simulink model "accController"  (R2022b)
settings: Solver=FixedStepAuto  StartTime=0.0  StopTime=120  FixedStep=tSample  RelTol=1e-3  EnableMultiTasking=on
PreLoadFcn:
  | if exist('tl_preloadfcn','file'), tl_preloadfcn(gcs,'22.1.0.27'); end
PostLoadFcn:
  | if exist('tl_postloadfcn','file'), tl_postloadfcn(gcs,'22.1.0.27'); end
InitFcn:
  | if exist('tlds_init','file'), tlds_init(gcs); end
StartFcn:
  | if exist('tlds_start','file'), tlds_start(gcs); end
StopFcn:
  | if exist('tlds_stop','file'), tlds_stop(gcs); end
model workspace (MAT data in the model file):
  obs_1 = 1
  obs_10 = 1
  obs_11 = 1
  obs_12 = 1
  obs_13 = 1
  obs_14 = 1
  obs_15 = 1
  obs_16 = 1
  obs_17 = 1
  obs_18 = 1
  obs_19 = 1
  obs_2 = 1
  obs_20 = 1
  obs_21 = 1
  obs_22 = 1
  obs_23 = 1
  obs_24 = 1
  obs_25 = 1
  obs_26 = 1
  obs_27 = 1
  obs_28 = 1
  obs_29 = 1
  obs_3 = 1
  obs_30 = 1
  obs_31 = 1
  obs_32 = 1
  obs_4 = 1
  obs_5 = 1
  obs_6 = 1
  obs_7 = 1
  obs_8 = 1
  obs_9 = 1
values from neighbouring files (symbols this model uses):
  pLutAccelMagnitude = [0, 0.1, 0.2, 0.3, 0.4, 0.5, 0.6, 0.7, 0.8, 0.9, 1,                        2.5, 3, 3.5, 4, 4.5, 5, 8, 12, 20]    [start.m]
  pLutAccelnSeverity = [0, 0.005, 0.05, 0.1, 0.15, 0.2, 0.3, 0.4, 0.6, 1, 3,                        5, 10, 17, 24, 32, 45, 60, 75, 100]    [start.m]
  pMaxAccAcceleration = 1.5    [start.m]
  pMaxAccDeacceleration = -1.5    [start.m]
  pMaxOperatingSpeed = 180    [start.m]
  pMinOperatingSpeed = 30    [start.m]
  tSample = 0.01    [start.m]
undefined symbols (not defined in the file or in its folder): Pedal, sigbuilder_block, vehicleDistanceRange
libraries: tllib x7
(part 1 of 5)
PreSaveFcn:
  | if exist('tl_presavefcn','file'), tl_presavefcn(gcs); end
CloseFcn:
  | if exist('tl_closefcn','file'), tl_closefcn(gcs); end
settings Model: TL_MAIN_DATA={'date',739002.69656854169,'advcodeopt',{'ExtendedBlockComments';'true'}}  DS_PROJECTFILE=accController.dd  TLVersion=22.1.0.27  TL_GLOBAL_LOGGING_MODE=4  PauseTimes=80.79  NumberOfSteps=100  Creator=developer  LastModifiedBy=developer
settings SolverCC: AlgebraicLoopSolver=TrustRegion
settings DataIOCC: LimitDataPoints=on  SaveFormat=Array  ReturnWorkspaceOutputs=off
settings OptimizationCC: BlockReduction=off  ConditionallyExecuteInputs=off  OptimizeBlockIOStorage=off  BufferReuse=off  GlobalBufferReuse=off  ExpressionFolding=off  LocalBlockOutputs=off  LifeSpan=inf  OptimizeDataStoreBuffers=off  BusAssignmentInplaceUpdate=off
settings DebuggingCC: UnconnectedInputMsg=warning  UnconnectedOutputMsg=warning  UnconnectedLineMsg=warning  BusObjectLabelMismatch=error  StrictBusMsg=ErrorOnBusTreatedAsVector  NonBusSignalsTreatedAsBus=error  SFUnexpectedBacktrackingDiag=warning  SFNoUnconditionalDefaultTransitionDiag=warning  SFMachineParentedDataDiag=warning  ArithmeticOperatorsInVariantConditions=warning
settings HardwareCC: ProdBitPerPointer=32  ProdBitPerSizeT=32  ProdBitPerPtrDiffT=32  ProdLargestAtomicFloat=None  ProdIntDivRoundTo=Undefined  ProdEndianess=Unspecified  ProdWordSize=32  ProdHWDeviceType=32-bit Generic
settings ModelReferenceCC: EnableRefExpFcnMdlSchedulingChecks=on  PropagateSignalLabelsOutOfModel=off
settings SFSimCC: SimUseLocalCustomCode=off  CustomCodeUndefinedFunction=UseInterfaceOnly
settings RTWCC: RTWUseLocalCustomCode=off
settings CodeAppCC: StateflowObjectComments=on
settings GRTTargetCC: TargetLangStandard=C89/C90 (ANSI)
settings ConfigComp: CovMetricSettings=dw  CovSaveCumulativeToWorkspaceVar=on  CovSaveSingleToWorkspaceVar=on  CovExternalEMLEnable=off

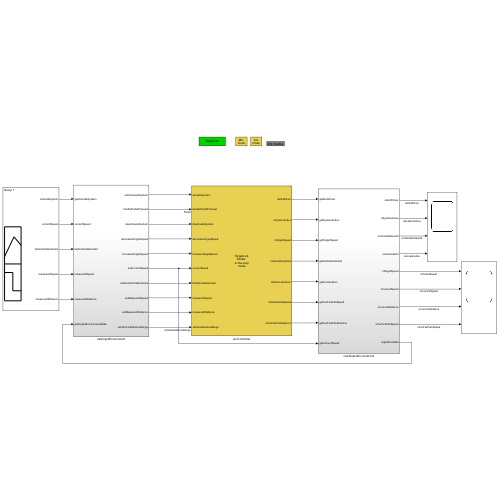
[thumbnail: Simulink's stored preview of the top-level diagram]
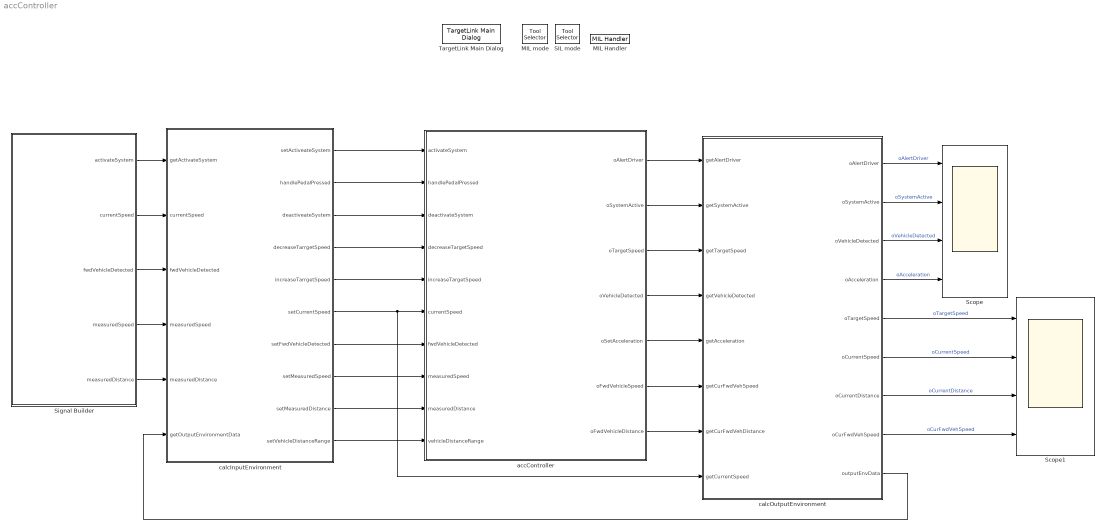
== system accController ==
  MIL Handler : tllib/MIL Handler  data={'date',730486}
      settings: SourceProductName=dSPACE TargetLink common blockset
  MIL mode : tllib/Tool Selector  Description=MIL\nmode  data={'date',730486}
      settings: SourceProductName=dSPACE TargetLink common blockset
  SIL mode : tllib/Tool Selector  Description=SIL\nmode  data={'date',730486}
      settings: SourceProductName=dSPACE TargetLink common blockset
  Scope : Scope  NumInputPorts=4
  Scope1 : Scope  NumInputPorts=4
  Signal Builder : Subsystem  Tag=STV Subsys  LoadFcn=sigbuilder_block('load');  StartFcn=sigbuilder_block('start');  StopFcn=sigbuilder_block('stop');  ClipboardFcn=sigbuilder_block('clipboard');  mask(Sigbuilder block){tuvar=[0:10]}
      mask help: Simulink:masks:SigbuilderBlock_MD
      mask init:
      | if ~strcmp(get_param(bdroot(gcbh),'SimulationStatus'),'stopped') tuvar = sigbuilder_block('maskInit'); end
      settings: CopyFcn=sigbuilder_block('copy');  DeleteFcn=sigbuilder_block('delete');  ModelCloseFcn=sigbuilder_block('modelClose');  PreSaveFcn=sigbuilder_block('preSave');  PauseFcn=sigbuilder_block('pause');  ContinueFcn=sigbuilder_block('continue');  NameChangeFcn=sigbuilder_block('namechange');  OpenFcn=sigbuilder_block('open',[133.5 114.75 1037.25 597 ]);  CloseFcn=sigbuilder_block('close');
      mask Display: plot(0, 0, 100, 100,[2, 2, 32, 32, 2], [68, 8, 8, 68, 68],[32, 2], [38, 38], [32, 19, 2],[53, 60, 44], [32, 17, 17, 2],[16, 16, 31, 31]);txt = getActiveGroup(gcbh);text(2, 100, txt,'verticalAlignment', 'top');
  TargetLink Main Dialog : tllib/TargetLink Main Dialog  data=[]
      settings: SourceProductName=dSPACE TargetLink common blockset
  accController : Subsystem  Tag=TargetLink Simulation Frame  mask(TL_SimFrame){}
      settings: CopyFcn=if exist('tl_copyfcn','file'), tl_copyfcn(gcbh); end  NameChangeFcn=if exist('tl_framenamechangefcn','file'), tl_framenamechangefcn(gcbh); end
      settings: OpenFcn=|
      | if exist('open_tlsubsystem','file')
      |    open_tlsubsystem(gcbh);
      | else
      |    tlsubsystem = ...
      |       find_system(gcb, ...
      |       'LookUnderMasks','on', ...
      |       'FollowLinks','on', ...
      |       'Tag','MIL Subsystem');
      |    open_system(tlsubsystem);
      | end
      mask Display: disp('TargetLink\nModel-\nin-the-loop\nmode')
  calcInputEnvironment : Subsystem
  calcOutputEnvironment : Subsystem
  wires:
  calcInputEnvironment/2(handlePedalPressed) -> accController/2(handlePedalPressed)
  calcInputEnvironment/10(setVehicleDistanceRange) -> accController/10(vehicleDistanceRange)
  accController/1(oAlertDriver) -> calcOutputEnvironment/1(getAlertDriver)
  calcInputEnvironment/9(setMeasuredDistance) -> accController/9(measuredDistance)
  accController/4(oVehicleDetected) -> calcOutputEnvironment/4(getVehicleDetected)
  calcInputEnvironment/6(setCurrentSpeed) -> calcOutputEnvironment/8(getCurrentSpeed), accController/6(currentSpeed)
  accController/5(oSetAcceleration) -> calcOutputEnvironment/5(getAcceleration)
  accController/6(oFwdVehicleSpeed) -> calcOutputEnvironment/6(getCurFwdVehSpeed)
  accController/7(oFwdVehicleDistance) -> calcOutputEnvironment/7(getCurFwdVehDistance)
  Signal Builder/1(activateSystem) -> calcInputEnvironment/1(getActivateSystem)
  Signal Builder/2(currentSpeed) -> calcInputEnvironment/2(currentSpeed)
  Signal Builder/3(fwdVehicleDetected) -> calcInputEnvironment/3(fwdVehicleDetected)
  Signal Builder/4(measuredSpeed) -> calcInputEnvironment/4(measuredSpeed)
  Signal Builder/5(measuredDistance) -> calcInputEnvironment/5(measuredDistance)
  accController/2(oSystemActive) -> calcOutputEnvironment/2(getSystemActive)
  accController/3(oTargetSpeed) -> calcOutputEnvironment/3(getTargetSpeed)
  calcInputEnvironment/3(deactiveateSystem) -> accController/3(deactivateSystem)
  calcInputEnvironment/4(decreaseTarrgetSpeed) -> accController/4(decreaseTargetSpeed)
  calcInputEnvironment/5(increaseTarrgetSpeed) -> accController/5(increaseTargetSpeed)
  calcOutputEnvironment/9(outputEnvData) -> calcInputEnvironment/6(getOutputEnvironmentData)
  calcInputEnvironment/7(setFwdVehicleDetected) -> accController/7(fwdVehicleDetected)
  calcInputEnvironment/8(setMeasuredSpeed) -> accController/8(measuredSpeed)
  calcInputEnvironment/1(setActiveateSystem) -> accController/1(activateSystem)
  calcOutputEnvironment/1(oAlertDriver) -> Scope/1  "oAlertDriver"
  calcOutputEnvironment/2(oSystemActive) -> Scope/2  "oSystemActive"
  calcOutputEnvironment/3(oVehicleDetected) -> Scope/3  "oVehicleDetected"
  calcOutputEnvironment/5(oTargetSpeed) -> Scope1/1  "oTargetSpeed"
  calcOutputEnvironment/6(oCurrentSpeed) -> Scope1/2  "oCurrentSpeed"
  calcOutputEnvironment/7(oCurrentDistance) -> Scope1/3  "oCurrentDistance"
  calcOutputEnvironment/8(oCurFwdVehSpeed) -> Scope1/4  "oCurFwdVehSpeed"
  calcOutputEnvironment/4(oAcceleration) -> Scope/4  "oAcceleration"

== system accController/Signal Builder ==
  Demux : Demux  Tag=STV Demux  Outputs=5
      settings: DisplayOption=none
  FromWs : FromWorkspace  Tag=STV FromWs  VariableName=tuvar
      SigBuilderData=|
      | common.afterFinalStr = 'Extrapolate'
      | common.sampleTime = 0
      | dataSet.timeRange = [0 120]
      | dataSet.name = 'Group 1'
      | sbobj.Groups.Name = 'Group 1'
      | sbobj.Groups.Signals(1).Name = 'activateSystem'
      | sbobj.Groups.Signals(1).XData = [0 12 12 13 13 120]
      | sbobj.Groups.Signals(1).YData = [0 0 1 1 0 0]
      | sbobj.Groups.Signals(2).Name = 'currentSpeed'
      | sbobj.Groups.Signals(2).XData = [0 12 120]
      | sbobj.Groups.Signals(2).YData = [0 135 135]
      | sbobj.Groups.Signals(3).Name = 'fwdVehicleDetected'
      | sbobj.Groups.Signals(3).XData = [0 20 20 120]
      | sbobj.Groups.Signals(3).YData = [0 0 1 1]
      | sbobj.Groups.Signals(4).Name = 'measuredSpeed'
      | sbobj.Groups.Signals(4).XData = [0 20 120]
      | sbobj.Groups.Signals(4).YData = [0 100 100]
      | sbobj.Groups.Signals(5).Name = 'measuredDistance'
      | sbobj.Groups.Signals(5).XData = [0 20 20 60 120]
      | sbobj.Groups.Signals(5).YData = [0 0 144 40 40]
      | sbobj.Groups.TimeRange = [0 120]
  activateSystem : Outport  Tag=STV Outport
  currentSpeed : Outport  Tag=STV Outport  Port=2
  fwdVehicleDetected : Outport  Tag=STV Outport  Port=3
  measuredSpeed : Outport  Tag=STV Outport  Port=4
  measuredDistance : Outport  Tag=STV Outport  Port=5
  wires:
  FromWs/1 -> Demux/1
  Demux/1 -> activateSystem/1
  Demux/2 -> currentSpeed/1
  Demux/3 -> fwdVehicleDetected/1
  Demux/4 -> measuredSpeed/1
  Demux/5 -> measuredDistance/1

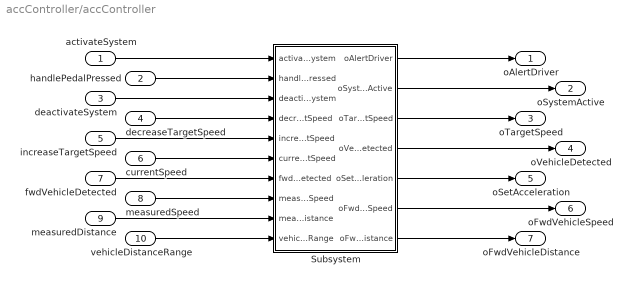
== system accController/accController ==
  activateSystem : Inport
  handlePedalPressed : Inport  Port=2  OutDataTypeStr=Enum: Pedal
  deactivateSystem : Inport  Port=3
  decreaseTargetSpeed : Inport  Port=4
  increaseTargetSpeed : Inport  Port=5
  currentSpeed : Inport  Port=6
  fwdVehicleDetected : Inport  Port=7
  measuredSpeed : Inport  Port=8
  measuredDistance : Inport  Port=9
  vehicleDistanceRange : Inport  Port=10  OutDataTypeStr=Enum: vehicleDistanceRange
  Subsystem : Subsystem  Tag=struct('sfcnName','accController_sf','subFunction','','srcSubsystem','')  mask(TL_Enable){}
      settings: OpenFcn=warndlg(get_param(gcb,'MaskHelp'),'Serious Warning');
      mask Help: This subsystem keeps the TargetLink subsystem (subsystem with TargetLink blocks for production code generation), and is needed for the TargetLink simulation frame to work properly. DO NOT DELETE OR MODIFY IT!
  oAlertDriver : Outport
  oSystemActive : Outport  Port=2
  oTargetSpeed : Outport  Port=3
  oVehicleDetected : Outport  Port=4
  oSetAcceleration : Outport  Port=5
  oFwdVehicleSpeed : Outport  Port=6
  oFwdVehicleDistance : Outport  Port=7
  wires:
  activateSystem/1 -> Subsystem/1(activateSystem)
  handlePedalPressed/1 -> Subsystem/2(handlePedalPressed)
  deactivateSystem/1 -> Subsystem/3(deactivateSystem)
  decreaseTargetSpeed/1 -> Subsystem/4(decreaseTargetSpeed)
  increaseTargetSpeed/1 -> Subsystem/5(increaseTargetSpeed)
  currentSpeed/1 -> Subsystem/6(currentSpeed)
  fwdVehicleDetected/1 -> Subsystem/7(fwdVehicleDetected)
  measuredSpeed/1 -> Subsystem/8(measuredSpeed)
  measuredDistance/1 -> Subsystem/9(measuredDistance)
  vehicleDistanceRange/1 -> Subsystem/10(vehicleDistanceRange)
  Subsystem/1(oAlertDriver) -> oAlertDriver/1
  Subsystem/2(oSystemActive) -> oSystemActive/1
  Subsystem/3(oTargetSpeed) -> oTargetSpeed/1
  Subsystem/4(oVehicleDetected) -> oVehicleDetected/1
  Subsystem/5(oSetAcceleration) -> oSetAcceleration/1
  Subsystem/6(oFwdVehicleSpeed) -> oFwdVehicleSpeed/1
  Subsystem/7(oFwdVehicleDistance) -> oFwdVehicleDistance/1

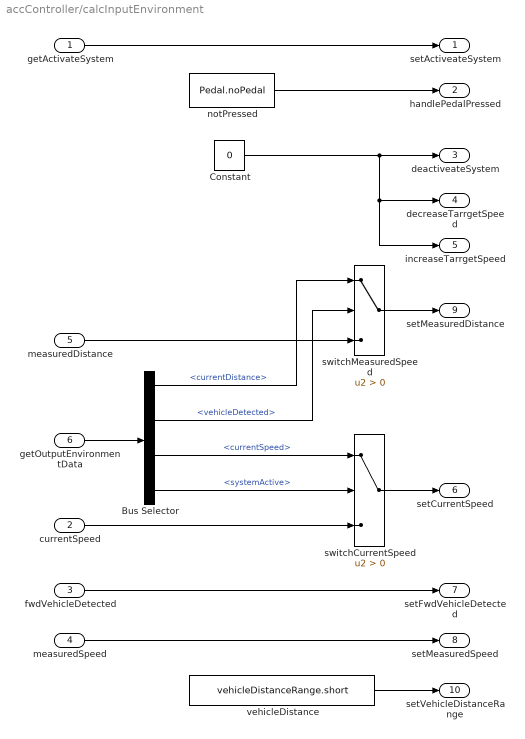
== system accController/calcInputEnvironment ==
  getActivateSystem : Inport
  currentSpeed : Inport  Port=2
  fwdVehicleDetected : Inport  Port=3
  measuredSpeed : Inport  Port=4
  measuredDistance : Inport  Port=5
  getOutputEnvironmentData : Inport  Port=6
  Bus Selector : BusSelector  OutputSignals=currentDistance,vehicleDetected,currentSpeed,systemActive
  Constant : Constant  Value=0
  notPressed : Constant  Value=Pedal.noPedal  OutDataTypeStr=Enum: Pedal
  switchCurrentSpeed : Switch  Criteria=u2 > Threshold  SaturateOnIntegerOverflow=off  InputSameDT=off
  switchMeasuredSpeed : Switch  Criteria=u2 > Threshold  SaturateOnIntegerOverflow=off  InputSameDT=off
  vehicleDistance : Constant  Value=vehicleDistanceRange.short  OutDataTypeStr=Enum: vehicleDistanceRange
  setActiveateSystem : Outport
  handlePedalPressed : Outport  Port=2
  deactiveateSystem : Outport  Port=3
  decreaseTarrgetSpeed : Outport  Port=4
  increaseTarrgetSpeed : Outport  Port=5
  setCurrentSpeed : Outport  Port=6
  setFwdVehicleDetected : Outport  Port=7
  setMeasuredSpeed : Outport  Port=8
  setMeasuredDistance : Outport  Port=9
  setVehicleDistanceRange : Outport  Port=10
  wires:
  getActivateSystem/1 -> setActiveateSystem/1
  vehicleDistance/1 -> setVehicleDistanceRange/1
  notPressed/1 -> handlePedalPressed/1
  Constant/1 -> increaseTarrgetSpeed/1, decreaseTarrgetSpeed/1, deactiveateSystem/1
  getOutputEnvironmentData/1 -> Bus Selector/1
  switchCurrentSpeed/1 -> setCurrentSpeed/1
  Bus Selector/4 -> switchCurrentSpeed/2  "<systemActive>"
  Bus Selector/3 -> switchCurrentSpeed/1  "<currentSpeed>"
  currentSpeed/1 -> switchCurrentSpeed/3
  fwdVehicleDetected/1 -> setFwdVehicleDetected/1
  Bus Selector/1 -> switchMeasuredSpeed/1  "<currentDistance>"
  Bus Selector/2 -> switchMeasuredSpeed/2  "<vehicleDetected>"
  measuredDistance/1 -> switchMeasuredSpeed/3
  switchMeasuredSpeed/1 -> setMeasuredDistance/1
  measuredSpeed/1 -> setMeasuredSpeed/1

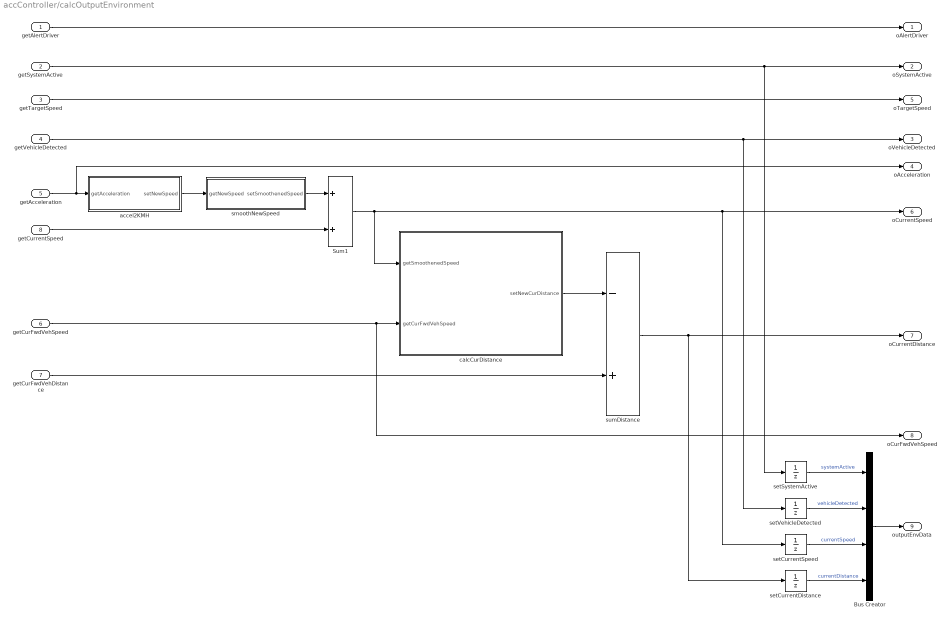
== system accController/calcOutputEnvironment ==
  getAlertDriver : Inport
  getSystemActive : Inport  Port=2
  getTargetSpeed : Inport  Port=3
  getVehicleDetected : Inport  Port=4
  getAcceleration : Inport  Port=5
  getCurFwdVehSpeed : Inport  Port=6
  getCurFwdVehDistance : Inport  Port=7
  getCurrentSpeed : Inport  Port=8
  Bus Creator : BusCreator  Inputs=4
  Sum1 : Sum
  accel2KMH : Subsystem
  calcCurDistance : Subsystem
  setCurrentDistance : UnitDelay  SampleTime=-1  HasFrameUpgradeWarning=on
  setCurrentSpeed : UnitDelay  SampleTime=-1  HasFrameUpgradeWarning=on
  setSystemActive : UnitDelay  SampleTime=-1  HasFrameUpgradeWarning=on
  setVehicleDetected : UnitDelay  SampleTime=-1  HasFrameUpgradeWarning=on
  smoothNewSpeed : Subsystem
  sumDistance : Sum  Inputs=-+
  oAlertDriver : Outport
  oSystemActive : Outport  Port=2
  oVehicleDetected : Outport  Port=3
  oAcceleration : Outport  Port=4
  oTargetSpeed : Outport  Port=5
  oCurrentSpeed : Outport  Port=6
  oCurrentDistance : Outport  Port=7
  oCurFwdVehSpeed : Outport  Port=8
  outputEnvData : Outport  Port=9
  wires:
  getAcceleration/1 -> oAcceleration/1, accel2KMH/1(getAcceleration)
  accel2KMH/1(setNewSpeed) -> smoothNewSpeed/1(getNewSpeed)
  smoothNewSpeed/1(setSmoothenedSpeed) -> Sum1/1
  Sum1/1 -> calcCurDistance/1(getSmoothenedSpeed), setCurrentSpeed/1, oCurrentSpeed/1
  getCurrentSpeed/1 -> Sum1/2
  getCurFwdVehSpeed/1 -> oCurFwdVehSpeed/1, calcCurDistance/2(getCurFwdVehSpeed)
  calcCurDistance/1(setNewCurDistance) -> sumDistance/1
  getCurFwdVehDistance/1 -> sumDistance/2
  sumDistance/1 -> oCurrentDistance/1, setCurrentDistance/1
  getAlertDriver/1 -> oAlertDriver/1
  getTargetSpeed/1 -> oTargetSpeed/1
  getSystemActive/1 -> oSystemActive/1, setSystemActive/1
  getVehicleDetected/1 -> oVehicleDetected/1, setVehicleDetected/1
  Bus Creator/1 -> outputEnvData/1
  setSystemActive/1 -> Bus Creator/1  "systemActive"
  setVehicleDetected/1 -> Bus Creator/2  "vehicleDetected"
  setCurrentSpeed/1 -> Bus Creator/3  "currentSpeed"
  setCurrentDistance/1 -> Bus Creator/4  "currentDistance"

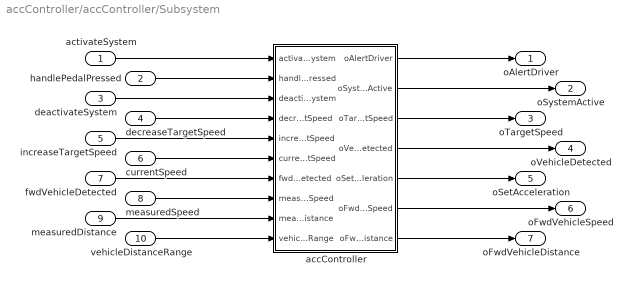
== system accController/accController/Subsystem ==
  activateSystem : Inport
  handlePedalPressed : Inport  Port=2
  deactivateSystem : Inport  Port=3
  decreaseTargetSpeed : Inport  Port=4
  increaseTargetSpeed : Inport  Port=5
  currentSpeed : Inport  Port=6
  fwdVehicleDetected : Inport  Port=7
  measuredSpeed : Inport  Port=8
  measuredDistance : Inport  Port=9
  vehicleDistanceRange : Inport  Port=10
  accController : Subsystem  Tag=MIL Subsystem  Description=a  LoadFcn=|
      | if exist('TargetLink.SimFrameHandler.TLSubsystem','class')
      |     TargetLink.SimFrameHandler.TLSubsystem.CreateWatchDog(gcbh);
      | end
      settings: AttributesFormatString=$ V-ECU simulation $\nUUID = ac35bcf0-8bf8-4691-a732-4e92aa29c2f7\nXCP-Port = \n  CopyFcn=if exist('tl_copyfcn','file'), tl_copyfcn(gcbh); end  NameChangeFcn=if exist('tl_namechangefcn','file'), tl_namechangefcn(gcbh); end  DestroyFcn=if exist('update_tl_main_dlg','file'), update_tl_main_dlg('TL_subs_display'); end
  oAlertDriver : Outport
  oSystemActive : Outport  Port=2
  oTargetSpeed : Outport  Port=3
  oVehicleDetected : Outport  Port=4
  oSetAcceleration : Outport  Port=5
  oFwdVehicleSpeed : Outport  Port=6
  oFwdVehicleDistance : Outport  Port=7
  wires:
  activateSystem/1 -> accController/1(activateSystem)
  handlePedalPressed/1 -> accController/2(handlePedalPressed)
  deactivateSystem/1 -> accController/3(deactivateSystem)
  decreaseTargetSpeed/1 -> accController/4(decreaseTargetSpeed)
  increaseTargetSpeed/1 -> accController/5(increaseTargetSpeed)
  currentSpeed/1 -> accController/6(currentSpeed)
  fwdVehicleDetected/1 -> accController/7(fwdVehicleDetected)
  measuredSpeed/1 -> accController/8(measuredSpeed)
  measuredDistance/1 -> accController/9(measuredDistance)
  vehicleDistanceRange/1 -> accController/10(vehicleDistanceRange)
  accController/1(oAlertDriver) -> oAlertDriver/1
  accController/2(oSystemActive) -> oSystemActive/1
  accController/3(oTargetSpeed) -> oTargetSpeed/1
  accController/4(oVehicleDetected) -> oVehicleDetected/1
  accController/5(oSetAcceleration) -> oSetAcceleration/1
  accController/6(oFwdVehicleSpeed) -> oFwdVehicleSpeed/1
  accController/7(oFwdVehicleDistance) -> oFwdVehicleDistance/1

== system accController/calcOutputEnvironment/accel2KMH ==
  getAcceleration : Inport
  acc2Speed : Product
  acc2Speed1 : Product
  ms2kmh : Constant  Value=3.6
  samplingTimeDiv : Constant  Value=tSample
  setNewSpeed : Outport
  wires:
  getAcceleration/1 -> acc2Speed/1
  samplingTimeDiv/1 -> acc2Speed/2
  acc2Speed/1 -> acc2Speed1/1
  ms2kmh/1 -> acc2Speed1/2
  acc2Speed1/1 -> setNewSpeed/1

== system accController/calcOutputEnvironment/calcCurDistance ==
  getSmoothenedSpeed : Inport
  getCurFwdVehSpeed : Inport  Port=2
  diffSpeed : Sum  Inputs=+-
  kmh2ms : Constant  Value=3.6
  kmh2msDiv : Product  Inputs=*/
  runDistance : Product
  samplingTimeDiv : Constant  Value=tSample
  setNewCurDistance : Outport
  wires:
  getSmoothenedSpeed/1 -> diffSpeed/1
  diffSpeed/1 -> kmh2msDiv/1
  kmh2ms/1 -> kmh2msDiv/2
  kmh2msDiv/1 -> runDistance/1
  samplingTimeDiv/1 -> runDistance/2
  runDistance/1 -> setNewCurDistance/1
  getCurFwdVehSpeed/1 -> diffSpeed/2

== system accController/calcOutputEnvironment/smoothNewSpeed ==
  getNewSpeed : Inport
  Abs : Abs  SaturateOnIntegerOverflow=off
  Sum : Sum
  chSpdThreshhold : Constant
  chSpeed : Switch  Criteria=u2 > Threshold  SaturateOnIntegerOverflow=off  InputSameDT=off
  changeSpeed : RelationalOperator  OutDataTypeStr=boolean  InputSameDT=off
  keepSpeed : Constant  Value=0
  resetUnitDelay : Switch  Threshold=1  SaturateOnIntegerOverflow=off  InputSameDT=off
  resetValue : Constant  Value=0
  sumSpeed : UnitDelay  SampleTime=-1  HasFrameUpgradeWarning=on
  setSmoothenedSpeed : Outport
  wires:
  changeSpeed/1 -> resetUnitDelay/2, chSpeed/2
  sumSpeed/1 -> Sum/1
  Sum/1 -> Abs/1, chSpeed/1, resetUnitDelay/3
  chSpdThreshhold/1 -> changeSpeed/2
  keepSpeed/1 -> chSpeed/3
  resetUnitDelay/1 -> sumSpeed/1
  resetValue/1 -> resetUnitDelay/1
  Abs/1 -> changeSpeed/1
  getNewSpeed/1 -> Sum/2
  chSpeed/1 -> setSmoothenedSpeed/1

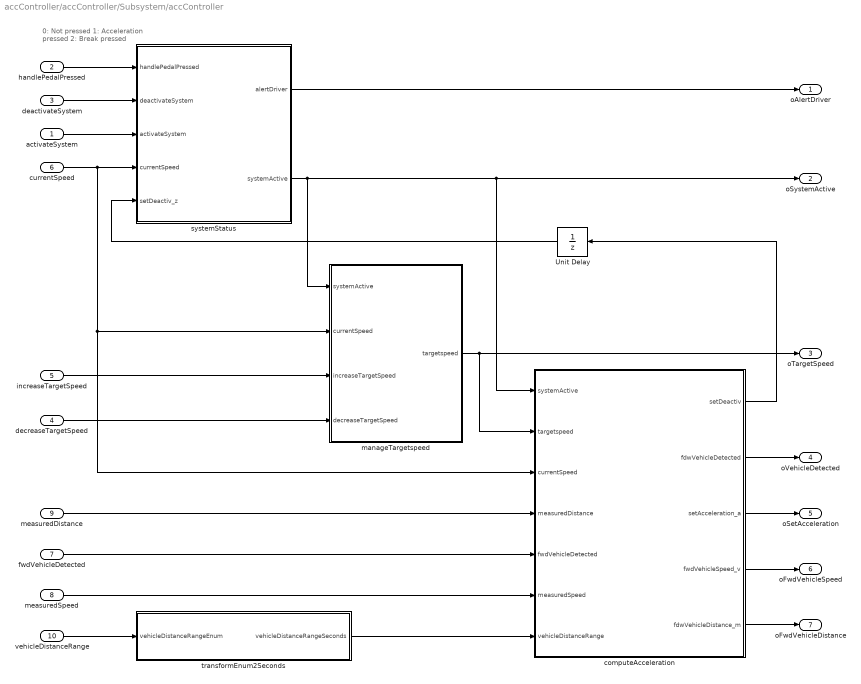
== system accController/accController/Subsystem/accController ==
  note: 0: Not pressed
      | 1: Acceleration pressed
      | 2: Break pressed
  activateSystem : Inport  PortDimensions=1  mask(TL_Inport){data={'output',{'variable','Inputs/activateSystem'},'date',737961.41640938655}}
      settings: CopyFcn=if exist('copy_tlblock','file')==2,copy_tlblock(gcbh);end  DeleteFcn=if exist('delete_tlblock','file')==2,delete_tlblock(gcbh);end  NameChangeFcn=if exist('rename_tlblock','file')==2,rename_tlblock(gcbh);end  OpenFcn=if exist('tl_open_blockdlg','file')==2,tl_open_blockdlg(gcbh);else,open_system(gcbh,'parameter');end
      mask Help: eval(['if exist(''tl_online_help'',''file'') == 2, tl_online_help(''Topic'',''TL_Inport''),else, web([''jar:file:///'',matlabroot,''/help/toolbox/simulink/help.jar!/slref/' lower(get_param(gcbh,'Blocktype')) '.html''], ''-helpbrowser''),end'])
      mask Display:
      | [x,y] = tlDrawBrandOnBlockIcon(gcbh);
      | plot(x,y);
  handlePedalPressed : Inport  Port=2  OutDataTypeStr=Enum: Pedal  PortDimensions=1  mask(TL_Inport){data={'output',{'variable','Inputs/handlePedalPressed'},'date',737961.41641082172}}
      settings: CopyFcn=if exist('copy_tlblock','file')==2,copy_tlblock(gcbh);end  DeleteFcn=if exist('delete_tlblock','file')==2,delete_tlblock(gcbh);end  NameChangeFcn=if exist('rename_tlblock','file')==2,rename_tlblock(gcbh);end  OpenFcn=if exist('tl_open_blockdlg','file')==2,tl_open_blockdlg(gcbh);else,open_system(gcbh,'parameter');end
      mask Help: eval(['if exist(''tl_online_help'',''file'') == 2, tl_online_help(''Topic'',''TL_Inport''),else, web([''jar:file:///'',matlabroot,''/help/toolbox/simulink/help.jar!/slref/' lower(get_param(gcbh,'Blocktype')) '.html''], ''-helpbrowser''),end'])
      mask Display:
      | [x,y] = tlDrawBrandOnBlockIcon(gcbh);
      | plot(x,y);
  deactivateSystem : Inport  Port=3  PortDimensions=1  mask(TL_Inport){data={'output',{'variable','Inputs/deactivateSystem'},'date',737961.41641125001}}
      settings: CopyFcn=if exist('copy_tlblock','file')==2,copy_tlblock(gcbh);end  DeleteFcn=if exist('delete_tlblock','file')==2,delete_tlblock(gcbh);end  NameChangeFcn=if exist('rename_tlblock','file')==2,rename_tlblock(gcbh);end  OpenFcn=if exist('tl_open_blockdlg','file')==2,tl_open_blockdlg(gcbh);else,open_system(gcbh,'parameter');end
      mask Help: eval(['if exist(''tl_online_help'',''file'') == 2, tl_online_help(''Topic'',''TL_Inport''),else, web([''jar:file:///'',matlabroot,''/help/toolbox/simulink/help.jar!/slref/' lower(get_param(gcbh,'Blocktype')) '.html''], ''-helpbrowser''),end'])
      mask Display:
      | [x,y] = tlDrawBrandOnBlockIcon(gcbh);
      | plot(x,y);
  decreaseTargetSpeed : Inport  Port=4  PortDimensions=1  mask(TL_Inport){data={'output',{'variable','Inputs/decreaseTargetSpeed'},'date',737961.41641188657}}
      settings: CopyFcn=if exist('copy_tlblock','file')==2,copy_tlblock(gcbh);end  DeleteFcn=if exist('delete_tlblock','file')==2,delete_tlblock(gcbh);end  NameChangeFcn=if exist('rename_tlblock','file')==2,rename_tlblock(gcbh);end  OpenFcn=if exist('tl_open_blockdlg','file')==2,tl_open_blockdlg(gcbh);else,open_system(gcbh,'parameter');end
      mask Help: eval(['if exist(''tl_online_help'',''file'') == 2, tl_online_help(''Topic'',''TL_Inport''),else, web([''jar:file:///'',matlabroot,''/help/toolbox/simulink/help.jar!/slref/' lower(get_param(gcbh,'Blocktype')) '.html''], ''-helpbrowser''),end'])
      mask Display:
      | [x,y] = tlDrawBrandOnBlockIcon(gcbh);
      | plot(x,y);
  increaseTargetSpeed : Inport  Port=5  PortDimensions=1  mask(TL_Inport){data={'output',{'variable','Inputs/increaseTargetSpeed'},'date',737961.41641219903}}
      settings: CopyFcn=if exist('copy_tlblock','file')==2,copy_tlblock(gcbh);end  DeleteFcn=if exist('delete_tlblock','file')==2,delete_tlblock(gcbh);end  NameChangeFcn=if exist('rename_tlblock','file')==2,rename_tlblock(gcbh);end  OpenFcn=if exist('tl_open_blockdlg','file')==2,tl_open_blockdlg(gcbh);else,open_system(gcbh,'parameter');end
      mask Help: eval(['if exist(''tl_online_help'',''file'') == 2, tl_online_help(''Topic'',''TL_Inport''),else, web([''jar:file:///'',matlabroot,''/help/toolbox/simulink/help.jar!/slref/' lower(get_param(gcbh,'Blocktype')) '.html''], ''-helpbrowser''),end'])
      mask Display:
      | [x,y] = tlDrawBrandOnBlockIcon(gcbh);
      | plot(x,y);
  currentSpeed : Inport  Port=6  PortDimensions=1  mask(TL_Inport){data={'output',{'variable','Inputs/currentSpeed'},'date',737961.41641256947}}
      settings: CopyFcn=if exist('copy_tlblock','file')==2,copy_tlblock(gcbh);end  DeleteFcn=if exist('delete_tlblock','file')==2,delete_tlblock(gcbh);end  NameChangeFcn=if exist('rename_tlblock','file')==2,rename_tlblock(gcbh);end  OpenFcn=if exist('tl_open_blockdlg','file')==2,tl_open_blockdlg(gcbh);else,open_system(gcbh,'parameter');end
      mask Help: eval(['if exist(''tl_online_help'',''file'') == 2, tl_online_help(''Topic'',''TL_Inport''),else, web([''jar:file:///'',matlabroot,''/help/toolbox/simulink/help.jar!/slref/' lower(get_param(gcbh,'Blocktype')) '.html''], ''-helpbrowser''),end'])
      mask Display:
      | [x,y] = tlDrawBrandOnBlockIcon(gcbh);
      | plot(x,y);
  fwdVehicleDetected : Inport  Port=7  PortDimensions=1  mask(TL_Inport){data={'output',{'variable','Inputs/fwdVehicleDetected'},'date',737961.41641273152}}
      settings: CopyFcn=if exist('copy_tlblock','file')==2,copy_tlblock(gcbh);end  DeleteFcn=if exist('delete_tlblock','file')==2,delete_tlblock(gcbh);end  NameChangeFcn=if exist('rename_tlblock','file')==2,rename_tlblock(gcbh);end  OpenFcn=if exist('tl_open_blockdlg','file')==2,tl_open_blockdlg(gcbh);else,open_system(gcbh,'parameter');end
      mask Help: eval(['if exist(''tl_online_help'',''file'') == 2, tl_online_help(''Topic'',''TL_Inport''),else, web([''jar:file:///'',matlabroot,''/help/toolbox/simulink/help.jar!/slref/' lower(get_param(gcbh,'Blocktype')) '.html''], ''-helpbrowser''),end'])
      mask Display:
      | [x,y] = tlDrawBrandOnBlockIcon(gcbh);
      | plot(x,y);
  measuredSpeed : Inport  Port=8  PortDimensions=1  mask(TL_Inport){data={'output',{'variable','Inputs/measuredSpeed'},'date',737961.41641285876}}
      settings: CopyFcn=if exist('copy_tlblock','file')==2,copy_tlblock(gcbh);end  DeleteFcn=if exist('delete_tlblock','file')==2,delete_tlblock(gcbh);end  NameChangeFcn=if exist('rename_tlblock','file')==2,rename_tlblock(gcbh);end  OpenFcn=if exist('tl_open_blockdlg','file')==2,tl_open_blockdlg(gcbh);else,open_system(gcbh,'parameter');end
      mask Help: eval(['if exist(''tl_online_help'',''file'') == 2, tl_online_help(''Topic'',''TL_Inport''),else, web([''jar:file:///'',matlabroot,''/help/toolbox/simulink/help.jar!/slref/' lower(get_param(gcbh,'Blocktype')) '.html''], ''-helpbrowser''),end'])
      mask Display:
      | [x,y] = tlDrawBrandOnBlockIcon(gcbh);
      | plot(x,y);
  measuredDistance : Inport  Port=9  PortDimensions=1  mask(TL_Inport){data={'output',{'variable','Inputs/measuredDistance'},'date',737961.41641302081}}
      settings: CopyFcn=if exist('copy_tlblock','file')==2,copy_tlblock(gcbh);end  DeleteFcn=if exist('delete_tlblock','file')==2,delete_tlblock(gcbh);end  NameChangeFcn=if exist('rename_tlblock','file')==2,rename_tlblock(gcbh);end  OpenFcn=if exist('tl_open_blockdlg','file')==2,tl_open_blockdlg(gcbh);else,open_system(gcbh,'parameter');end
      mask Help: eval(['if exist(''tl_online_help'',''file'') == 2, tl_online_help(''Topic'',''TL_Inport''),else, web([''jar:file:///'',matlabroot,''/help/toolbox/simulink/help.jar!/slref/' lower(get_param(gcbh,'Blocktype')) '.html''], ''-helpbrowser''),end'])
      mask Display:
      | [x,y] = tlDrawBrandOnBlockIcon(gcbh);
      | plot(x,y);
  vehicleDistanceRange : Inport  Port=10  OutDataTypeStr=Enum: vehicleDistanceRange  PortDimensions=1  mask(TL_Inport){data={'output',{'variable','Inputs/handleDistanceRange'},'date',737961.41641317133}}
      settings: CopyFcn=if exist('copy_tlblock','file')==2,copy_tlblock(gcbh);end  DeleteFcn=if exist('delete_tlblock','file')==2,delete_tlblock(gcbh);end  NameChangeFcn=if exist('rename_tlblock','file')==2,rename_tlblock(gcbh);end  OpenFcn=if exist('tl_open_blockdlg','file')==2,tl_open_blockdlg(gcbh);else,open_system(gcbh,'parameter');end
      mask Help: eval(['if exist(''tl_online_help'',''file'') == 2, tl_online_help(''Topic'',''TL_Inport''),else, web([''jar:file:///'',matlabroot,''/help/toolbox/simulink/help.jar!/slref/' lower(get_param(gcbh,'Blocktype')) '.html''], ''-helpbrowser''),end'])
      mask Display:
      | [x,y] = tlDrawBrandOnBlockIcon(gcbh);
      | plot(x,y);
  Unit Delay : UnitDelay  SampleTime=-1  HasFrameUpgradeWarning=on  mask(TL_UnitDelay){data={'output',{'type','Bool'},'state',{'type','Bool'},'date',739002.69656527776}}
      settings: CopyFcn=if exist('copy_tlblock','file')==2,copy_tlblock(gcbh);end  DeleteFcn=if exist('delete_tlblock','file')==2,delete_tlblock(gcbh);end  NameChangeFcn=if exist('rename_tlblock','file')==2,rename_tlblock(gcbh);end  OpenFcn=if exist('tl_open_blockdlg','file')==2,tl_open_blockdlg(gcbh);else,open_system(gcbh,'parameter');end
      mask Help: eval(['if exist(''tl_online_help'',''file'') == 2, tl_online_help(''Topic'',''TL_UnitDelay''),else, web([''jar:file:///'',matlabroot,''/help/toolbox/simulink/help.jar!/slref/' lower(get_param(gcbh,'Blocktype')) '.html''], ''-helpbrowser''),end'])
      mask Display:
      | [x,y] = tlDrawBrandOnBlockIcon(gcbh);
      | plot(x,y);
  computeAcceleration : Subsystem  TreatAsAtomicUnit=on
  manageTargetspeed : Subsystem
  systemStatus : Subsystem  TreatAsAtomicUnit=on
  transformEnum2Seconds : Subsystem
  oAlertDriver : Outport  PortDimensions=1  mask(TL_Outport){data={'output',{'variable','Outputs/oAlertDriver'},'date',737961.41641591431}}
      settings: CopyFcn=if exist('copy_tlblock','file')==2,copy_tlblock(gcbh);end  DeleteFcn=if exist('delete_tlblock','file')==2,delete_tlblock(gcbh);end  NameChangeFcn=if exist('rename_tlblock','file')==2,rename_tlblock(gcbh);end  OpenFcn=if exist('tl_open_blockdlg','file')==2,tl_open_blockdlg(gcbh);else,open_system(gcbh,'parameter');end
      mask Help: eval(['if exist(''tl_online_help'',''file'') == 2, tl_online_help(''Topic'',''TL_Outport''),else, web([''jar:file:///'',matlabroot,''/help/toolbox/simulink/help.jar!/slref/' lower(get_param(gcbh,'Blocktype')) '.html''], ''-helpbrowser''),end'])
      mask Display:
      | [x,y] = tlDrawBrandOnBlockIcon(gcbh);
      | plot(x,y);
  oSystemActive : Outport  Port=2  PortDimensions=1  mask(TL_Outport){data={'output',{'variable','Outputs/oSystemActive'},'date',737961.41641619208}}
      settings: CopyFcn=if exist('copy_tlblock','file')==2,copy_tlblock(gcbh);end  DeleteFcn=if exist('delete_tlblock','file')==2,delete_tlblock(gcbh);end  NameChangeFcn=if exist('rename_tlblock','file')==2,rename_tlblock(gcbh);end  OpenFcn=if exist('tl_open_blockdlg','file')==2,tl_open_blockdlg(gcbh);else,open_system(gcbh,'parameter');end
      mask Help: eval(['if exist(''tl_online_help'',''file'') == 2, tl_online_help(''Topic'',''TL_Outport''),else, web([''jar:file:///'',matlabroot,''/help/toolbox/simulink/help.jar!/slref/' lower(get_param(gcbh,'Blocktype')) '.html''], ''-helpbrowser''),end'])
      mask Display:
      | [x,y] = tlDrawBrandOnBlockIcon(gcbh);
      | plot(x,y);
  oTargetSpeed : Outport  Port=3  PortDimensions=1  mask(TL_Outport){data={'output',{'variable','Outputs/oTargetSpeed'},'date',737961.41641635413}}
      settings: CopyFcn=if exist('copy_tlblock','file')==2,copy_tlblock(gcbh);end  DeleteFcn=if exist('delete_tlblock','file')==2,delete_tlblock(gcbh);end  NameChangeFcn=if exist('rename_tlblock','file')==2,rename_tlblock(gcbh);end  OpenFcn=if exist('tl_open_blockdlg','file')==2,tl_open_blockdlg(gcbh);else,open_system(gcbh,'parameter');end
      mask Help: eval(['if exist(''tl_online_help'',''file'') == 2, tl_online_help(''Topic'',''TL_Outport''),else, web([''jar:file:///'',matlabroot,''/help/toolbox/simulink/help.jar!/slref/' lower(get_param(gcbh,'Blocktype')) '.html''], ''-helpbrowser''),end'])
      mask Display:
      | [x,y] = tlDrawBrandOnBlockIcon(gcbh);
      | plot(x,y);
  oVehicleDetected : Outport  Port=4  PortDimensions=1  mask(TL_Outport){data={'output',{'variable','Outputs/oVehicledetected'},'date',737961.41641649301}}
      settings: CopyFcn=if exist('copy_tlblock','file')==2,copy_tlblock(gcbh);end  DeleteFcn=if exist('delete_tlblock','file')==2,delete_tlblock(gcbh);end  NameChangeFcn=if exist('rename_tlblock','file')==2,rename_tlblock(gcbh);end  OpenFcn=if exist('tl_open_blockdlg','file')==2,tl_open_blockdlg(gcbh);else,open_system(gcbh,'parameter');end
      mask Help: eval(['if exist(''tl_online_help'',''file'') == 2, tl_online_help(''Topic'',''TL_Outport''),else, web([''jar:file:///'',matlabroot,''/help/toolbox/simulink/help.jar!/slref/' lower(get_param(gcbh,'Blocktype')) '.html''], ''-helpbrowser''),end'])
      mask Display:
      | [x,y] = tlDrawBrandOnBlockIcon(gcbh);
      | plot(x,y);
  oSetAcceleration : Outport  Port=5  PortDimensions=1  mask(TL_Outport){data={'output',{'variable','Outputs/oSetAcceleration'},'date',737961.4164167014}}
      settings: CopyFcn=if exist('copy_tlblock','file')==2,copy_tlblock(gcbh);end  DeleteFcn=if exist('delete_tlblock','file')==2,delete_tlblock(gcbh);end  NameChangeFcn=if exist('rename_tlblock','file')==2,rename_tlblock(gcbh);end  OpenFcn=if exist('tl_open_blockdlg','file')==2,tl_open_blockdlg(gcbh);else,open_system(gcbh,'parameter');end
      mask Help: eval(['if exist(''tl_online_help'',''file'') == 2, tl_online_help(''Topic'',''TL_Outport''),else, web([''jar:file:///'',matlabroot,''/help/toolbox/simulink/help.jar!/slref/' lower(get_param(gcbh,'Blocktype')) '.html''], ''-helpbrowser''),end'])
      mask Display:
      | [x,y] = tlDrawBrandOnBlockIcon(gcbh);
      | plot(x,y);
  oFwdVehicleSpeed : Outport  Port=6  PortDimensions=1  mask(TL_Outport){data={'output',{'variable','Outputs/oFwdVehicleSpeed'},'date',737961.41641687497}}
      settings: CopyFcn=if exist('copy_tlblock','file')==2,copy_tlblock(gcbh);end  DeleteFcn=if exist('delete_tlblock','file')==2,delete_tlblock(gcbh);end  NameChangeFcn=if exist('rename_tlblock','file')==2,rename_tlblock(gcbh);end  OpenFcn=if exist('tl_open_blockdlg','file')==2,tl_open_blockdlg(gcbh);else,open_system(gcbh,'parameter');end
      mask Help: eval(['if exist(''tl_online_help'',''file'') == 2, tl_online_help(''Topic'',''TL_Outport''),else, web([''jar:file:///'',matlabroot,''/help/toolbox/simulink/help.jar!/slref/' lower(get_param(gcbh,'Blocktype')) '.html''], ''-helpbrowser''),end'])
      mask Display:
      | [x,y] = tlDrawBrandOnBlockIcon(gcbh);
      | plot(x,y);
  oFwdVehicleDistance : Outport  Port=7  PortDimensions=1  mask(TL_Outport){data={'output',{'variable','Outputs/oFwdVehicleDistance'},'date',737961.41641704866}}
      settings: CopyFcn=if exist('copy_tlblock','file')==2,copy_tlblock(gcbh);end  DeleteFcn=if exist('delete_tlblock','file')==2,delete_tlblock(gcbh);end  NameChangeFcn=if exist('rename_tlblock','file')==2,rename_tlblock(gcbh);end  OpenFcn=if exist('tl_open_blockdlg','file')==2,tl_open_blockdlg(gcbh);else,open_system(gcbh,'parameter');end
      mask Help: eval(['if exist(''tl_online_help'',''file'') == 2, tl_online_help(''Topic'',''TL_Outport''),else, web([''jar:file:///'',matlabroot,''/help/toolbox/simulink/help.jar!/slref/' lower(get_param(gcbh,'Blocktype')) '.html''], ''-helpbrowser''),end'])
      mask Display:
      | [x,y] = tlDrawBrandOnBlockIcon(gcbh);
      | plot(x,y);
  wires:
  handlePedalPressed/1 -> systemStatus/1(handlePedalPressed)
  deactivateSystem/1 -> systemStatus/2(deactivateSystem)
  activateSystem/1 -> systemStatus/3(activateSystem)
  manageTargetspeed/1(targetspeed) -> oTargetSpeed/1, computeAcceleration/2(targetspeed)
  increaseTargetSpeed/1 -> manageTargetspeed/3(increaseTargetSpeed)
  decreaseTargetSpeed/1 -> manageTargetspeed/4(decreaseTargetSpeed)
  fwdVehicleDetected/1 -> computeAcceleration/5(fwdVehicleDetected)
  measuredSpeed/1 -> computeAcceleration/6(measuredSpeed)
  measuredDistance/1 -> computeAcceleration/4(measuredDistance)
  currentSpeed/1 -> computeAcceleration/3(currentSpeed), manageTargetspeed/2(currentSpeed), systemStatus/4(currentSpeed)
  systemStatus/1(alertDriver) -> oAlertDriver/1
  systemStatus/2(systemActive) -> manageTargetspeed/1(systemActive), computeAcceleration/1(systemActive), oSystemActive/1
  vehicleDistanceRange/1 -> transformEnum2Seconds/1(vehicleDistanceRangeEnum)
  transformEnum2Seconds/1(vehicleDistanceRangeSeconds) -> computeAcceleration/7(vehicleDistanceRange)
  computeAcceleration/1(setDeactiv) -> Unit Delay/1
  computeAcceleration/2(fdwVehicleDetected) -> oVehicleDetected/1
  computeAcceleration/3(setAcceleration_a) -> oSetAcceleration/1
  computeAcceleration/4(fwdVehicleSpeed_v) -> oFwdVehicleSpeed/1
  computeAcceleration/5(fdwVehicleDistance_m) -> oFwdVehicleDistance/1
  Unit Delay/1 -> systemStatus/5(setDeactiv_z)
